simulink model "SuperTwistingSMC"  (R2015b)
settings: Solver=VariableStepAuto  StartTime=0.0  StopTime=10.0  RelTol=1e-3
values from neighbouring files (symbols this model uses):
  B = 5    [SMC_Mass_Spring_Damper.m]
  K = 2    [SMC_Mass_Spring_Damper.m]
  M = 2    [SMC_Mass_Spring_Damper.m]
libraries: simulink x1
settings Model: Creator=mathi  LastModifiedBy=mathi

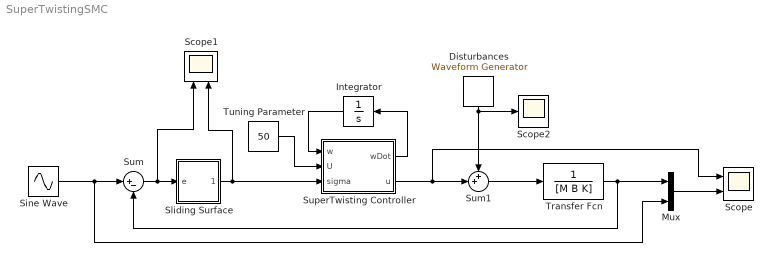
== system SuperTwistingSMC ==
  Disturbances : simulink/Sources/Waveform Generator  OutMin=[]  OutMax=[]  OutDataTypeStr=double  SelectedSignal=1  Signals=2+2*sin(1,3,0)+sin(1,5,0)  BlockNames=MultiportSwitch_82285e9e5ef0486  SampleTime=0.001
  Integrator : Integrator
  Mux : Mux  Inputs=2
  Scope : Scope  NumInputPorts=2
  Scope1 : Scope  NumInputPorts=2
  Scope2 : Scope
  Sine Wave : Sin  Frequency=2  SampleTime=0
  "Sliding Surface " : Subsystem
  Sum : Sum  Inputs=|+-
  Sum1 : Sum  Inputs=++|
  SuperTwisting Controller : MATLAB Function  TreatAsAtomicUnit=on
  Transfer Fcn : TransferFcn  Denominator=[M B K]
  Tuning Parameter : Constant  Value=50
  wires:
  Sine Wave/1 -> Mux/2, Sum/1
  Transfer Fcn/1 -> Mux/1, Sum/2
  Mux/1 -> Scope/2
  "Sliding Surface "/1(Sigma) -> SuperTwisting Controller/3(sigma), Scope1/2
  SuperTwisting Controller/1(wDot) -> Integrator/1
  Integrator/1 -> SuperTwisting Controller/1(w)
  Tuning Parameter/1 -> SuperTwisting Controller/2(U)
  Sum/1 -> Scope1/1, "Sliding Surface "/1(e)
  SuperTwisting Controller/2(u) -> Scope/1, Sum1/2
  Sum1/1 -> Transfer Fcn/1
  Disturbances/1 -> Sum1/1, Scope2/1

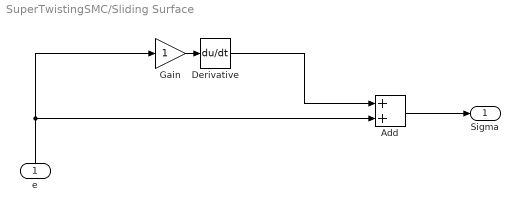
== system SuperTwistingSMC/Sliding Surface  ==
  e : Inport
  Add : Sum
  Derivative : Derivative
  Gain : Gain
  Sigma : Outport
  wires:
  Gain/1 -> Derivative/1
  Derivative/1 -> Add/1
  Add/1 -> Sigma/1
  e/1 -> Add/2, Gain/1

== matlab function SuperTwistingSMC/SuperTwisting Controller ==
  data: w input; U input; wDot output; u output; sigma input
function [wDot,u] = fcn(w,U,sigma)

lambda = sqrt(U);
W = 1.1*U;

u = lambda*sqrt(abs(sigma))*sign(sigma) + w;
wDot = W*sign(sigma);
